simulink model "thermal_model_lumped"  (R2016a)
settings: Solver=ode4  StartTime=0.0  StopTime=Tfinal  FixedStep=Ts  RelTol=1e-3
values from neighbouring files (symbols this model uses):
  PGaN = 8    [thermal_lumped.m]
  Rth_hs = (Rth_base*Rth_fin)./(Rth_base+Rth_fin)    [thermal_calc_forjournal.m]    (also in thermal_lumped.m = 0.05*(k))
  Rth_jc = 0.5    [thermal_lumped.m]
  Rth_pad = Rth_pa + 2*Rth_tim    (= 2.85185185185)    [thermal_lumped.m]
  Rth_pcb = 3.39    [thermal_calc.m]    (also in thermal_calc_forjournal.m; thermal_lumped.m)
  Ta = 40    [thermal_lumped.m]
  Ts = 1e-3    (= 0.001)    [thermal_lumped.m]
undefined symbols (not defined in the file or in its folder): Lload
libraries: powerlib x40
settings Model: Creator=ugurm  LastModifiedBy=mesutto
settings DataIOCC: LimitDataPoints=on  SaveFormat=Array
settings DebuggingCC: UnderspecifiedInitializationDetection=Classic  MergeDetectMultiDrivingBlocksExec=none  SolverPrmCheckMsg=warning  StateNameClashWarn=warning
settings HardwareCC: ProdBitPerPointer=32  ProdLargestAtomicFloat=None  ProdIntDivRoundTo=Undefined  ProdEndianess=Unspecified  ProdWordSize=32  ProdHWDeviceType=32-bit Generic
settings ModelReferenceCC: PropagateSignalLabelsOutOfModel=off
settings ConfigComp: CovModelRefEnable=Off

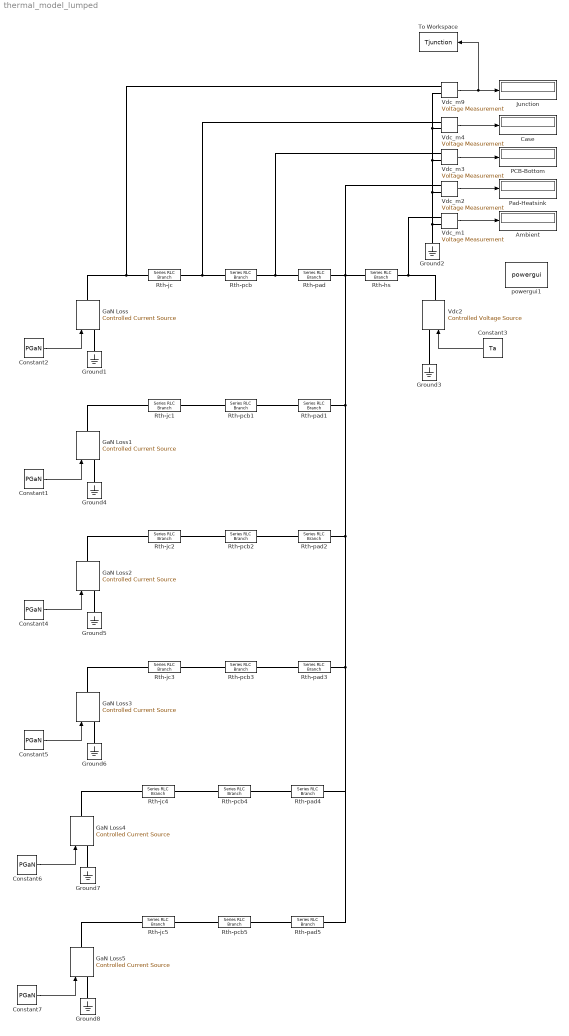
== system thermal_model_lumped ==
  Ambient : Display
  Case : Display
  Constant{1..2,4..7} (6 alike) : Constant  Value=PGaN
  Constant3 : Constant  Value=Ta
  GaN Loss{,1..5} (6 alike) : powerlib/Electrical Sources/Controlled Current Source  Initialize=on  Source_Type=AC  Amplitude=0  Phase=0  Frequency=0  Measurements=None
  Ground{1..8} (8 alike) : powerlib/Elements/Ground  LConnTagsString=a
  Junction : Display
  PCB-Bottom : Display
  Pad-Heatsink : Display
  Rth-hs : powerlib/Elements/Series RLC Branch  LConnTagsString=__new0  RConnTagsString=__new0  BranchType=R  Resistance=Rth_hs  Inductance=Lload  SetiL0=off  InitialCurrent=0  Capacitance=1e-6  Setx0=off  InitialVoltage=0  Measurements=None
  Rth-jc{,1..5} (6 alike) : powerlib/Elements/Series RLC Branch  LConnTagsString=__new0  RConnTagsString=__new0  BranchType=R  Resistance=Rth_jc  Inductance=Lload  SetiL0=off  InitialCurrent=0  Capacitance=1e-6  Setx0=off  InitialVoltage=0  Measurements=None
  Rth-pad{,1..5} (6 alike) : powerlib/Elements/Series RLC Branch  LConnTagsString=__new0  RConnTagsString=__new0  BranchType=R  Resistance=Rth_pad  Inductance=Lload  SetiL0=off  InitialCurrent=0  Capacitance=1e-6  Setx0=off  InitialVoltage=0  Measurements=None
  Rth-pcb{,1..5} (6 alike) : powerlib/Elements/Series RLC Branch  LConnTagsString=__new0  RConnTagsString=__new0  BranchType=R  Resistance=Rth_pcb  Inductance=Lload  SetiL0=off  InitialCurrent=0  Capacitance=1e-6  Setx0=off  InitialVoltage=0  Measurements=None
  To Workspace : ToWorkspace  VariableName=Tjunction  SampleTime=-1
  Vdc2 : powerlib/Electrical Sources/Controlled Voltage Source  Initialize=off  Source_Type=DC  Amplitude=200  Phase=0  Frequency=0  Measurements=None
  Vdc_m{1..4,9} (5 alike) : powerlib/Measurements/Voltage Measurement  PhasorSimulation=off  OutputType=Complex  PSBequivalent=0
  powergui1 : powerlib/powergui  Priority=1  SimulationMode=Discrete  SolverType=Tustin  SampleTime=Ts  frequency=60  SPID=off  DisableSnubberDevices=off  DisableRonSwitches=off  DisableVfSwitches=off  SwTol=0  DisplayEquations=off  Interpol=off  ExternalGateDelay=off  methode=off  Ts=0  FunctionMessages=off  echomessages=off  HookPort=off  EnableUseOfTLC=off  x0status=blocks  frequencyindice=0  Pbase=100e6  ErrMax=1e-4  Iterations=50  UnitsV=kV  UnitsW=MW  buscounter=0  RestoreLinks=warning  ResistiveCurrentMeasurement=off  Frange=[0:2:500]  Ylog=off  Xlog=on  ShowGrid=off  save=off  variable=ZData  structure=Vdc  ZoomFFT=off  StartTime=0.04  cycles=5  DisplayStyle=5  fundamental=50  FreqAxis=off  MaxFrequency=30000  frequencyindicesteady=1  RmsSteady=1  display=off
  wires:
  Constant2/1 -> GaN Loss/1
  Constant3/1 -> Vdc2/1
  Vdc_m4/1 -> Case/1
  Vdc_m3/1 -> PCB-Bottom/1
  Vdc_m2/1 -> Pad-Heatsink/1
  Vdc_m1/1 -> Ambient/1
  Constant1/1 -> GaN Loss1/1
  Constant4/1 -> GaN Loss2/1
  Constant5/1 -> GaN Loss3/1
  Constant6/1 -> GaN Loss4/1
  Constant7/1 -> GaN Loss5/1
  Vdc_m9/1 -> To Workspace/1, Junction/1
  connections:
  GaN Loss/LConn1 -- Ground1/LConn1
  Rth-jc/LConn1 -- Vdc_m9/LConn1 -- GaN Loss/RConn1
  Rth-pcb/LConn1 -- Vdc_m4/LConn1 -- Rth-jc/RConn1
  Rth-pad/LConn1 -- Vdc_m3/LConn1 -- Rth-pcb/RConn1
  Rth-hs/LConn1 -- Rth-pad5/RConn1 -- Rth-pad4/RConn1 -- Rth-pad3/RConn1 -- Rth-pad2/RConn1 -- Rth-pad1/RConn1 -- Vdc_m2/LConn1 -- Rth-pad/RConn1
  Vdc2/RConn1 -- Vdc_m1/LConn1 -- Rth-hs/RConn1
  Ground2/LConn1 -- Vdc_m1/LConn2 -- Vdc_m2/LConn2 -- Vdc_m3/LConn2 -- Vdc_m4/LConn2 -- Vdc_m9/LConn2
  Ground3/LConn1 -- Vdc2/LConn1
  Rth-jc1/LConn1 -- GaN Loss1/RConn1
  Rth-pcb1/LConn1 -- Rth-jc1/RConn1
  Rth-pad1/LConn1 -- Rth-pcb1/RConn1
  GaN Loss1/LConn1 -- Ground4/LConn1
  Rth-jc2/LConn1 -- GaN Loss2/RConn1
  GaN Loss2/LConn1 -- Ground5/LConn1
  Rth-pad2/LConn1 -- Rth-pcb2/RConn1
  Rth-pcb2/LConn1 -- Rth-jc2/RConn1
  Rth-jc3/LConn1 -- GaN Loss3/RConn1
  GaN Loss3/LConn1 -- Ground6/LConn1
  Rth-pad3/LConn1 -- Rth-pcb3/RConn1
  Rth-pcb3/LConn1 -- Rth-jc3/RConn1
  Rth-jc5/LConn1 -- GaN Loss5/RConn1
  GaN Loss4/LConn1 -- Ground7/LConn1
  Rth-pad4/LConn1 -- Rth-pcb4/RConn1
  Rth-jc4/LConn1 -- GaN Loss4/RConn1
  Rth-pcb4/LConn1 -- Rth-jc4/RConn1
  GaN Loss5/LConn1 -- Ground8/LConn1
  Rth-pad5/LConn1 -- Rth-pcb5/RConn1
  Rth-pcb5/LConn1 -- Rth-jc5/RConn1
